simulink model "week2_problem4"  (R2020b)
settings: Solver=VariableStepAuto  StartTime=0.0  StopTime=10.0  RelTol=1e-3
model workspace (MAT data in the model file):
  J = Simulink.Parameter
  J.Value = 3.2284e-06
  J.DataType = 'auto'
  J.Dimensions = [1 1]
  K = Simulink.Parameter
  K.Value = 0.0274
  K.DataType = 'auto'
  K.Dimensions = [1 1]
  L = Simulink.Parameter
  L.Value = 2.75e-06
  L.DataType = 'auto'
  L.Dimensions = [1 1]
  R = Simulink.Parameter
  R.Value = 4
  R.DataType = 'auto'
  R.Dimensions = [1 1]
  b = Simulink.Parameter
  b.Value = 3.5077e-06
  b.DataType = 'auto'
  b.Dimensions = [1 1]
settings Model: Creator=gokul  LastModifiedBy=gokul

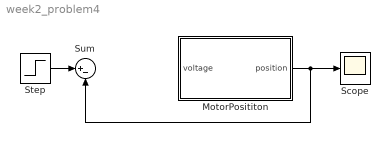
== system week2_problem4 ==
  MotorPosititon : Subsystem
  Scope : Scope
  Step : Step  SampleTime=0
  Sum : Sum  Inputs=|+-
  wires:
  Step/1 -> Sum/1
  MotorPosititon/1(position) -> Sum/2, Scope/1

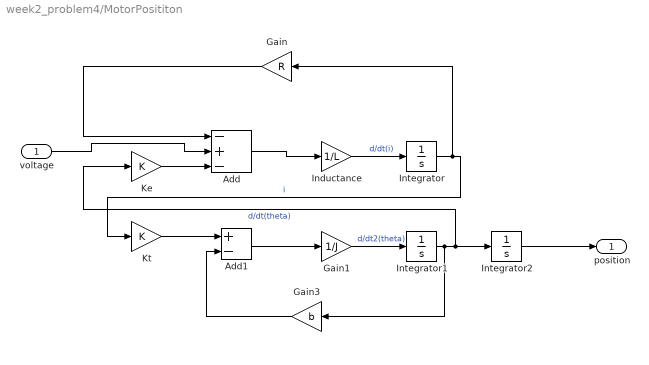
== system week2_problem4/MotorPosititon ==
  voltage : Inport
  Add : Sum  Inputs=-+-
  Add1 : Sum  Inputs=+-
  Gain : Gain  Gain=R
  Gain1 : Gain  Gain=1/J
  Gain3 : Gain  Gain=b
  Inductance : Gain  Gain=1/L
  Integrator : Integrator
  Integrator1 : Integrator
  Integrator2 : Integrator
  Ke : Gain  Gain=K
  Kt : Gain  Gain=K
  position : Outport
  wires:
  Integrator1/1 -> Gain3/1, Ke/1, Integrator2/1  "d/dt(theta)"
  Integrator/1 -> Gain/1, Kt/1  "i"
  Gain1/1 -> Integrator1/1  "d/dt2(theta)"
  voltage/1 -> Add/2
  Gain3/1 -> Add1/2
  Add1/1 -> Gain1/1
  Ke/1 -> Add/3
  Kt/1 -> Add1/1
  Inductance/1 -> Integrator/1  "d/dt(i)"
  Add/1 -> Inductance/1
  Gain/1 -> Add/1
  Integrator2/1 -> position/1
